simulink model "pfb_fir_generic_test_sim4"  (R2012b)
settings: Solver=VariableStepDiscrete  StartTime=0.0  StopTime=10.0  RelTol=1e-3
model workspace (MAT data in the model file):
  synci = [0 1 2 3 4 5 6 7 8 9 10 11 ... (589826 elements, 294913x2)]
  din0 = [0 1 2 3 4 5 6 7 8 9 10 11 ... (73730 elements, 36865x2)]
  din1 = [0 1 2 3 4 5 6 7 8 9 10 11 ... (73730 elements, 36865x2)]
  din2 = [0 1 2 3 4 5 6 7 8 9 10 11 ... (73730 elements, 36865x2)]
  din3 = [0 1 2 3 4 5 6 7 8 9 10 11 ... (73730 elements, 36865x2)]
  din4 = [0 1 2 3 4 5 6 7 8 9 10 11 ... (73730 elements, 36865x2)]
  din5 = [0 1 2 3 4 5 6 7 8 9 10 11 ... (73730 elements, 36865x2)]
  din6 = [0 1 2 3 4 5 6 7 8 9 10 11 ... (73730 elements, 36865x2)]
  din7 = [0 1 2 3 4 5 6 7 8 9 10 11 ... (73730 elements, 36865x2)]
libraries: xbsIndex_r4 x5323, casper_library_delays x1
(part 1 of 23)
settings Model: Creator=andrew  LastModifiedBy=andrew

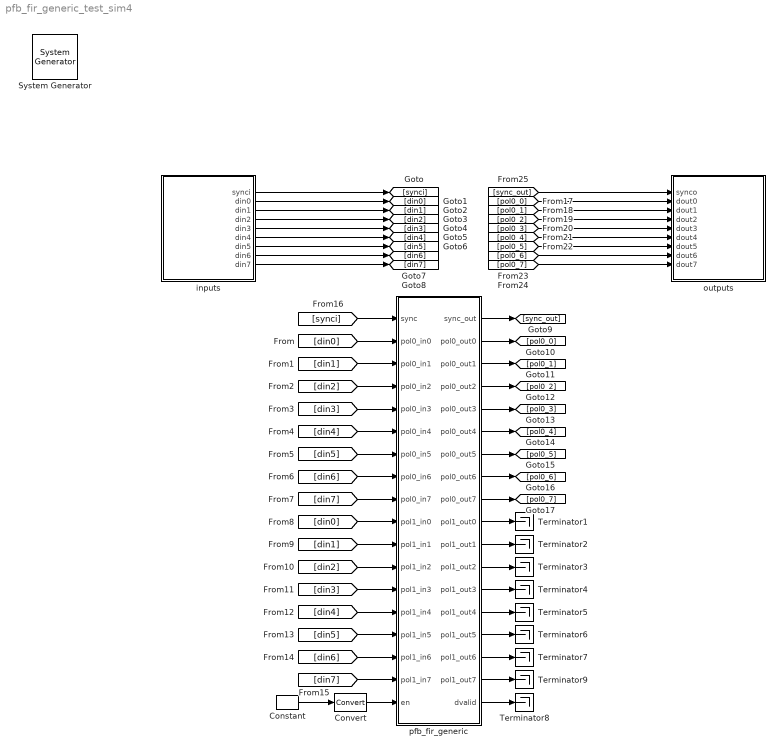
== system pfb_fir_generic_test_sim4 ==
  " System Generator" : xbsIndex_r4/ System Generator  Tag=genX  xilinxfamily=Kintex7  part=xc7k325t  speed=-3  package=fbg676  synthesis_tool=XST  clock_wrapper=Clock Enables  directory=./netlist  proj_type=Project Navigator  Synth_file=XST Defaults  Impl_file=ISE Defaults  testbench=off  simulink_period=1  sysclk_period=10  dcm_input_clock_period=10  incr_netlist=off  trim_vbits=Everywhere in SubSystem  dbl_ovrd=According to Block Masks  core_generation=According to Block Masks  run_coregen=off  deprecated_control=off  eval_field=0  block_type=sysgen
  Constant : xbsIndex_r4/Constant  const=1  gui_display_data_type=Boolean  arith_type=Boolean  n_bits=16  bin_pt=14  preci_type=Single  exp_width=8  frac_width=24  explicit_period=on  period=1  equ=P=C  opselect=C  inp2=PCIN>>17  opr=+  inp1=P  carry=CIN  dbl_ovrd=off  block_type=constant
  Convert : xbsIndex_r4/Convert  gui_display_data_type=Boolean  arith_type=Boolean  n_bits=16  bin_pt=14  float_type=Single  exp_bits=8  fraction_bits=24  quantization=Truncate  overflow=Wrap  en=off  latency=0  dbl_ovrd=off  pipeline=off  block_type=convert
  Terminator{1..9} (9 alike) : Terminator
  inputs : Subsystem
  outputs : Subsystem
  pfb_fir_generic : Subsystem  Tag=casper:pfb_fir_generic  AncestorBlock=casper_library_pfbs/pfb_fir_generic  mask(pfb_fir_generic){n_streams=2, PFBSize=13, TotalTaps=4, WindowType=hamming, n_inputs=3, BitWidthIn=10, BitWidthOut=18, CoeffBitWidth=18, complex=off, async=on, add_latency=2, mult_latency=3, bram_latency=7, fan_latency=9, conv_latency=3, quantization=Round  (unbiased: +/- Inf), fwidth=1, coeffs_bram_optimization=Speed, delays_bram_optimization=Speed}
      mask prompts: n_streams "Number input streams?"; PFBSize "Size of PFB: (2^? pnts)"; TotalTaps "Total Number of Taps:"; WindowType "Windowing Function:"; n_inputs "Number of Simultaneous Inputs: (2^?)"; BitWidthIn "Input Bitwidth:"; BitWidthOut "Output Bitwidth:"; CoeffBitWidth "Coefficient Bitwidth:"; complex "Complex data inputs"; async "Asynchronous operation"; add_latency "Add Latency"; mult_latency "Mult Latency"; bram_latency "BRAM Latency"; fan_latency "Fanout Latency"; conv_latency "Convert latency"; quantization "Quantization Behavior"; fwidth "Bin Width Scaling (normal=1)"; coeffs_bram_optimization "Coefficient BRAMs optimization"; delays_bram_optimization "Delay BRAMs optimization"
      mask init:
      | pfb_fir_generic_init(gcb, ...
      |     'n_streams', n_streams, ...
      |     'PFBSize', PFBSize, ...
      |     'TotalTaps', TotalTaps, ...
      |     'WindowType', WindowType, ...
      |     'n_inputs', n_inputs, ...
      |     'complex', complex, ...
      |     'BitWidthIn', BitWidthIn, ...
      |     'BitWidthOut', BitWidthOut, ...
      |     'CoeffBitWidth', CoeffBitWidth, ...
      |     'async', async, ...
      |     'add_latency', add_latency, ...
      |     'mult_latency', mult_latency, ...
      |     'bram_latency', bram_latency, ...
      |     'fan_latency', fan_latency, ...
      |     'conv_latency', conv_latency, ...
      |     'quantization', quantization, ...
      |     'fwidth', fwidth, ...
      |     'coeffs_bram_optimization', coeffs_bram_optimization, ...
      |     'delays_bram_optimization', delays_bram_optimization);
      mask Callback TotalTaps:
      | %num_taps = eval(get_param(gcb, 'TotalTaps'));
      | %old_vec = eval(get_param(gcb, 'mult_spec'));
      | 
      | %vec = 2.*ones(1,num_taps);
      | %old_size = length(old_vec);
      | 
      | %if(old_size <= num_taps),
      | %   new_size = old_size;
      | %else,
      | %    new_size = num_taps;
      | %end
      | 
      | %for n = 1:new_size, vec(n) = old_vec(n); end
      | %set_param(gcb, 'mult_spec', mat2str(vec));
      mask TypeOptions WindowType: bartlett | barthannwin | blackman | blackmanharris | bohamwin | chebwin | flattopwin | gausswin | hamming | hann | kaiser | nuttallwin | parzenwin | rectwin | tukeywin | triang | userwindow
      mask TypeOptions quantization: Truncate | Round  (unbiased: +/- Inf) | Round  (unbiased: Even Values)
      mask Callback fwidth:
      | %num_taps = eval(get_param(gcb, 'TotalTaps'));
      | %old_vec = eval(get_param(gcb, 'mult_spec'));
      | 
      | %vec = 2.*ones(1,num_taps);
      | %old_size = length(old_vec);
      | 
      | %if(old_size <= num_taps),
      | %    new_size = old_size;
      | %else,
      | %    new_size = num_taps;
      | %end
      | 
      | %for n = 1:new_size, vec(n) = old_vec(n); end
      | %set_param(gcb, 'mult_spec', mat2str(vec));
      mask TypeOptions coeffs_bram_optimization: Area | Speed
      mask TypeOptions delays_bram_optimization: Area | Speed
  wires:
  inputs/1(synci) -> [synci]
  inputs/2(din0) -> [din0]
  inputs/3(din1) -> [din1]
  inputs/4(din2) -> [din2]
  inputs/5(din3) -> [din3]
  inputs/6(din4) -> [din4]
  inputs/7(din5) -> [din5]
  inputs/8(din6) -> [din6]
  inputs/9(din7) -> [din7]
  Constant/1 -> Convert/1
  [pol0_7] -> outputs/9(dout7)
  [pol0_6] -> outputs/8(dout6)
  [pol0_5] -> outputs/7(dout5)
  [pol0_4] -> outputs/6(dout4)
  [pol0_3] -> outputs/5(dout3)
  [pol0_2] -> outputs/4(dout2)
  [pol0_1] -> outputs/3(dout1)
  [pol0_0] -> outputs/2(dout0)
  [sync_out] -> outputs/1(synco)
  pfb_fir_generic/10(pol1_out0) -> Terminator1/1
  pfb_fir_generic/11(pol1_out1) -> Terminator2/1
  pfb_fir_generic/12(pol1_out2) -> Terminator3/1
  pfb_fir_generic/13(pol1_out3) -> Terminator4/1
  pfb_fir_generic/14(pol1_out4) -> Terminator5/1
  pfb_fir_generic/15(pol1_out5) -> Terminator6/1
  pfb_fir_generic/16(pol1_out6) -> Terminator7/1
  pfb_fir_generic/18(dvalid) -> Terminator8/1
  Convert/1 -> pfb_fir_generic/18(en)
  [din0] -> pfb_fir_generic/2(pol0_in0)
  [din1] -> pfb_fir_generic/3(pol0_in1)
  [din2] -> pfb_fir_generic/4(pol0_in2)
  [din3] -> pfb_fir_generic/5(pol0_in3)
  [din4] -> pfb_fir_generic/6(pol0_in4)
  [din5] -> pfb_fir_generic/7(pol0_in5)
  [din6] -> pfb_fir_generic/8(pol0_in6)
  [din7] -> pfb_fir_generic/9(pol0_in7)
  [din0] -> pfb_fir_generic/10(pol1_in0)
  [din1] -> pfb_fir_generic/11(pol1_in1)
  [din2] -> pfb_fir_generic/12(pol1_in2)
  [din3] -> pfb_fir_generic/13(pol1_in3)
  [din4] -> pfb_fir_generic/14(pol1_in4)
  [din5] -> pfb_fir_generic/15(pol1_in5)
  [din6] -> pfb_fir_generic/16(pol1_in6)
  [din7] -> pfb_fir_generic/17(pol1_in7)
  [synci] -> pfb_fir_generic/1(sync)
  pfb_fir_generic/9(pol0_out7) -> [pol0_7]
  pfb_fir_generic/8(pol0_out6) -> [pol0_6]
  pfb_fir_generic/7(pol0_out5) -> [pol0_5]
  pfb_fir_generic/6(pol0_out4) -> [pol0_4]
  pfb_fir_generic/5(pol0_out3) -> [pol0_3]
  pfb_fir_generic/4(pol0_out2) -> [pol0_2]
  pfb_fir_generic/3(pol0_out1) -> [pol0_1]
  pfb_fir_generic/2(pol0_out0) -> [pol0_0]
  pfb_fir_generic/1(sync_out) -> [sync_out]
  pfb_fir_generic/17(pol1_out7) -> Terminator9/1
